simulink model "buck_dcm_vs1"  (Simulink 9.1)
settings: Solver=VariableStepAuto  StartTime=0.0  StopTime=0.0375  RelTol=1e-3
settings Model: Creator=xiaodong  LastModifiedBy=xiaodong
settings DataIOCC: SaveFormat=Dataset
settings OptimizationCC: LifeSpan=auto
settings DebuggingCC: UnderspecifiedInitializationDetection=Simplified  MergeDetectMultiDrivingBlocksExec=error  SFUnexpectedBacktrackingDiag=error  SFNoUnconditionalDefaultTransitionDiag=error  SFExecutionAtInitializationDiag=warning
settings HardwareCC: ProdBitPerPointer=64  ProdBitPerSizeT=64  ProdBitPerPtrDiffT=64  ProdLargestAtomicFloat=Float  ProdIntDivRoundTo=Zero  ProdEndianess=LittleEndian  ProdWordSize=64  ProdHWDeviceType=Intel->x86-64 (Windows64)
settings ModelReferenceCC: PropagateSignalLabelsOutOfModel=on
settings CodeAppCC: StateflowObjectComments=off
settings GRTTargetCC: TargetLangStandard=C99 (ISO)  CombineOutputUpdateFcns=on  GRTInterface=off
settings ConfigComp: CovMetricSettings=dwe  CovHtmlReporting=off  CovSaveCumulativeToWorkspaceVar=off  CovSaveSingleToWorkspaceVar=off  CovExternalEMLEnable=on

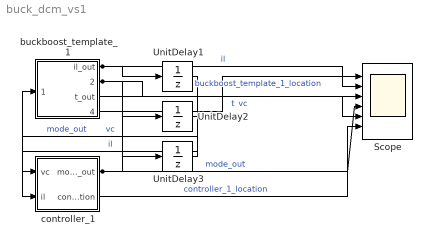
== system buck_dcm_vs1 ==
  Scope : Scope  NumInputPorts=6
  UnitDelay1 : UnitDelay  SampleTime=1/500000
  UnitDelay2 : UnitDelay  SampleTime=1/500000
  UnitDelay3 : UnitDelay  SampleTime=1/500000
  buckboost_template_1 : Stateflow chart  TreatAsAtomicUnit=on
  controller_1 : Stateflow chart  TreatAsAtomicUnit=on
  wires:
  buckboost_template_1/4(buckboost_template_1_location) -> Scope/1  "buckboost_template_1_location"
  buckboost_template_1/1(il_out) -> Scope/2, UnitDelay1/1  "il"
  UnitDelay1/1 -> controller_1/2(il)  "il"
  buckboost_template_1/3(t_out) -> Scope/3  "t"
  controller_1/1(mode_out_out) -> Scope/4, UnitDelay2/1  "mode_out"
  UnitDelay2/1 -> buckboost_template_1/1(mode_out)  "mode_out"
  buckboost_template_1/2(vc_out) -> Scope/5, UnitDelay3/1  "vc"
  UnitDelay3/1 -> controller_1/1(vc)  "vc"
  controller_1/2(controller_1_location) -> Scope/6  "controller_1_location"

== stateflow chart controller_1 ==
  settings: updateMethod=DISCRETE  sampleTime=1/50000
  state controller_11
    entry:
    mode_out_out=mode_out;
    controller_1_location  =1;
  state controller_12
    entry:
    mode_out_out=mode_out;
    controller_1_location  =2;
  controller_11 -> controller_11 [order 2] : [vc < VcH]
  controller_12 -> controller_12 [order 1] : [vc > VcL]
  controller_11 -> controller_12 [order 1] : [vc >= VcH]
      | {mode_out = 1.0;}
  controller_12 -> controller_11 [order 2] : [vc <= VcL]
      | {mode_out = 2.0;}
  (default) -> controller_11 : {mode_out = 2.0;}
  data: vc input double; mode_out_out output double; mode_out local double; il input double; controller_1_location output double; tmax constant double =0.0375; VcH constant double =12.1; Vs constant double =24; VcL constant double =11.9
  data vc settings: updateMethod=SF_CONTINUOUS_TIME_DATA
  data mode_out settings: updateMethod=SF_CONTINUOUS_TIME_DATA
  data il settings: updateMethod=SF_CONTINUOUS_TIME_DATA

== stateflow chart buckboost_template_1 ==
  settings: updateMethod=CONTINUOUS
  state charging
    du:
    il_dot = a00c * il + a01c * vc + b0c * Vs;
    vc_dot = a10c * il + a11c * vc + b1c * Vs;
    t_dot = 1.0;
    il_out=il;
    vc_out=vc;
    t_out=t;
    buckboost_template_1_location =1;
  state discharging
    du:
    il_dot = a00o * il + a01o * vc + b0o * Vs;
    vc_dot = a10o * il + a11o * vc + b1o * Vs;
    t_dot = 1.0;
    il_out=il;
    vc_out=vc;
    t_out=t;
    buckboost_template_1_location =2;
  state dcm
    du:
    il_dot = 0.0;
    vc_dot = a11o * vc + b1o * Vs;
    t_dot = 1.0;
    il_out=il;
    vc_out=vc;
    t_out=t;
    buckboost_template_1_location =3;
  charging -> discharging : [ mode_out == 1.0]
  discharging -> dcm [order 2] : [il <= 0.0]
  (default) -> charging : {il = 0.0;
      | vc = 0.0;
      | t = 0.0;}
  discharging -> charging [order 1] : [ mode_out == 2.0]
  dcm -> charging : [ mode_out == 2.0]
  data: il_out output double; il local double; vc_out output double; vc local double; t_out output double; t local double; mode_out input double; buckboost_template_1_location output double; b0o constant double =0; a01o constant double =-377.3585; b1o constant double =0; a00o constant double =-196.2264; a11o constant double =-45.4545; a10o constant double =454.5455; tmax constant double =0.0375; a01c constant double =-377.3585; a00c constant double =-271.6981; a11c constant double =-45.4545; a10c constant double =454.5455; b0c constant double =377.3585; b1c constant double =0; bounds constant double =1000; VcH constant double =12.1; Vs constant double =24; VcL constant double =11.9
  data il settings: updateMethod=SF_CONTINUOUS_TIME_DATA
  data vc settings: updateMethod=SF_CONTINUOUS_TIME_DATA
  data t settings: updateMethod=SF_CONTINUOUS_TIME_DATA
  data mode_out settings: updateMethod=SF_CONTINUOUS_TIME_DATA
